simulink library "csu_smp_sensonor_messsage_processing_lib"  (R2014b)
settings: Solver=ode45  StartTime=0.0  StopTime=10.0  RelTol=1e-3
libraries: simulink x1, util_info_lib x1, util_common_lib x1
settings Model: Creator=escrane  LastModifiedBy=mstewart

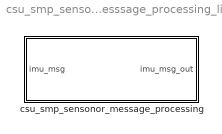
== system csu_smp_sensonor_messsage_processing_lib ==
  csu_smp_sensonor_message_processing : Subsystem

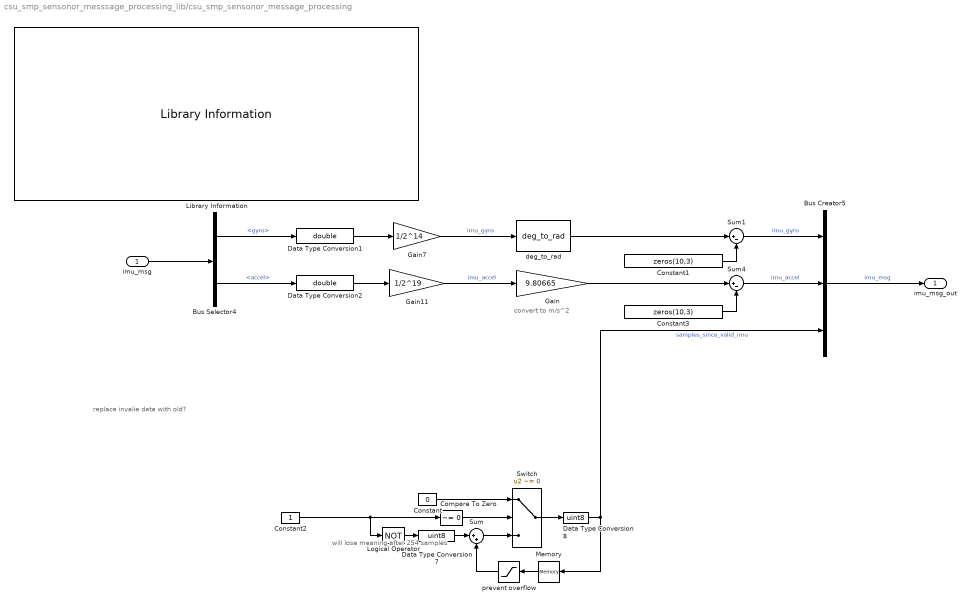
== system csu_smp_sensonor_messsage_processing_lib/csu_smp_sensonor_message_processing ==
  note: will lose meaning after 254 samples
  note: replace invalie data with old?
  note: convert to m/s^2
  imu_msg : Inport
  Bus Creator5 : BusCreator  Inputs=3
  Bus Selector4 : BusSelector  OutputSignals=gyro,accel
  Compare To Zero : simulink/Logic and Bit Operations/Compare To Zero  relop=~=  OutDataTypeStr=boolean
  Constant : Constant  Value=0  OutDataTypeStr=uint8
  Constant1 : Constant  Value=zeros(10,3)  OutDataTypeStr=double
  Constant2 : Constant  OutDataTypeStr=uint8
  Constant3 : Constant  Value=zeros(10,3)  OutDataTypeStr=double
  Data Type Conversion1 : DataTypeConversion  OutDataTypeStr=double
  Data Type Conversion2 : DataTypeConversion  OutDataTypeStr=double
  Data Type Conversion7 : DataTypeConversion  OutDataTypeStr=uint8
  Data Type Conversion8 : DataTypeConversion  OutDataTypeStr=uint8
  Gain : Gain  Gain=9.80665
  Gain11 : Gain  Gain=1/2^19  OutDataTypeStr=double
  Gain7 : Gain  Gain=1/2^14  OutDataTypeStr=double
  Library Information : util_info_lib/Library Information  owner='escrane'
  Logical Operator : Logic  Operator=NOT  AllPortsSameDT=off  OutDataTypeStr=boolean
  Memory : Memory  X0=uint8(0)  InheritSampleTime=on
  Sum : Sum  Inputs=|++
  Sum1 : Sum  Inputs=|+-
  Sum4 : Sum  Inputs=|+-
  Switch : Switch  Criteria=u2 ~= 0
  deg_to_rad : util_common_lib/deg_to_rad  SystemSampleTime=-1
  prevent overflow : Saturate  UpperLimit=254  LowerLimit=0
  imu_msg_out : Outport
  wires:
  deg_to_rad/1 -> Sum1/1
  Gain/1 -> Sum4/1
  Bus Selector4/2 -> Data Type Conversion2/1  "<accel>"
  Bus Selector4/1 -> Data Type Conversion1/1  "<gyro>"
  Constant1/1 -> Sum1/2
  Constant3/1 -> Sum4/2
  Gain11/1 -> Gain/1  "imu_accel"
  Gain7/1 -> deg_to_rad/1  "imu_gyro"
  Data Type Conversion8/1 -> Memory/1, Bus Creator5/3  "samples_since_valid_imu"
  Switch/1 -> Data Type Conversion8/1
  prevent overflow/1 -> Sum/2
  Logical Operator/1 -> Data Type Conversion7/1
  Data Type Conversion7/1 -> Sum/1
  Compare To Zero/1 -> Switch/2
  Sum/1 -> Switch/3
  Constant/1 -> Switch/1
  Memory/1 -> prevent overflow/1
  Constant2/1 -> Compare To Zero/1, Logical Operator/1
  Sum4/1 -> Bus Creator5/2  "imu_accel"
  Sum1/1 -> Bus Creator5/1  "imu_gyro"
  Data Type Conversion2/1 -> Gain11/1
  Data Type Conversion1/1 -> Gain7/1
  imu_msg/1 -> Bus Selector4/1
  Bus Creator5/1 -> imu_msg_out/1  "imu_msg"
